simulink library "inp"  (R2021b)
settings: Solver=VariableStepAuto  StartTime=0.0  StopTime=10.0  RelTol=1e-3
undefined symbols (not defined in the file): C_TASK_5MS_S, FALSE, KINP_AcoreReadyToSlp_flg_ovrdflg, KINP_AcoreReadyToSlp_flg_ovrdval, KINP_AllowMovThd_OTA_enum_ovrdflg, KINP_AllowMovThd_OTA_enum_ovrdval, KINP_APSAngleTarget_Deg_ovrdflg, KINP_APSAngleTarget_Deg_ovrdval, KINP_APSDecReq_mps2_ovrdflg, KINP_APSDecReq_mps2_ovrdval, KINP_APSDecReqA_flg_ovrdflg, KINP_APSDecReqA_flg_ovrdval, KINP_APSDFLL_cm_ovrdflg, KINP_APSDFLL_cm_ovrdval, KINP_APSDFLR_cm_ovrdflg, KINP_APSDFLR_cm_ovrdval, KINP_APSDRLL_cm_ovrdflg, KINP_APSDRLL_cm_ovrdval, KINP_APSDRLR_cm_ovrdflg, KINP_APSDRLR_cm_ovrdval, KINP_APSExitCondition_enum_ovrdflg, KINP_APSExitCondition_enum_ovrdval, KINP_APSHWVer_enum_ovrdflg, KINP_APSHWVer_enum_ovrdval, KINP_APSProgressPCT_pct_ovrdflg, KINP_APSProgressPCT_pct_ovrdval, KINP_APSReq_enum_ovrdflg, KINP_APSReq_enum_ovrdval, KINP_APSRQDisplay_enum_ovrdflg, KINP_APSRQDisplay_enum_ovrdval, KINP_APSRqEPASCtrl_flg_ovrdflg, KINP_APSRqEPASCtrl_flg_ovrdval, KINP_APSShiftPosnReq_enum_ovrdval, KINP_APSShiftPosnReq_enum_ovrflg, KINP_APSSpeedCMD_kph_ovrdval, KINP_APSSpeedCMD_kph_ovrflg, KINP_APSStaSystem_enum_ovrdflg, KINP_APSStaSystem_enum_ovrdval, KINP_APSSWVer_enum_ovrdflg, KINP_APSSWVer_enum_ovrdval, KINP_APSVMCReqA_flg_ovrdval, KINP_APSVMCReqA_flg_ovrflg, KINP_APSVRqEPASCtrl_flg_ovrdflg, KINP_APSVRqEPASCtrl_flg_ovrdval, KINP_AuxBattVolmV_mV_ovrdflg, KINP_AuxBattVolmV_mV_ovrdval, KINP_CAASSta_enum_ovrdflg, KINP_CAASSta_enum_ovrdval, KINP_CAASVMCReqA_flg_ovrdval, KINP_CAASVMCReqA_flg_ovrflg, KINP_Chime_enum_ovrdflg, KINP_Chime_enum_ovrdval, KINP_ClearDTCcmd_flg_ovrdflg, KINP_ClearDTCcmd_flg_ovrdval, KINP_EvccAplusPwrUpReq_flg_ovrdflg, KINP_EvccAplusPwrUpReq_flg_ovrdval, KINP_LFID_raw_ovrdval, KINP_LFID_raw_ovrflg, KINP_LRID_raw_ovrdval, KINP_MemOffsetAccX_raw16_ovrdflg ... (+118)
libraries: FVT_lib x595, hcu_lib x1
(part 15 of 27)

== system inp/INP/CAN2/SignalCheck/IVI6 ==
  BHAL_outputs : Inport
  inp_CanValid_bus : Inport  Port=2
  IVILocatedSTA : FVT_lib/inp/can_signal_template  SystemSampleTime=-1  VariantActivationTime=update diagram  Latency=0  AutoFrameSizeCalculation=off
      link override defval: Value=KINP_IVILocatedSTA_enum_defval
      link override fftdec: Value=KINP_IVILocatedSTA_enum_fftdec
      link override fftinc: Value=KINP_IVILocatedSTA_enum_fftinc
      link override fftlim: Value=KINP_IVILocatedSTA_enum_fftlim
      link override invalid: Value=KINP_IVILocatedSTA_enum_invalid
      link override ovrdflg: Value=KINP_IVILocatedSTA_enum_ovrdflg
      link override ovrdval: Value=KINP_IVILocatedSTA_enum_ovrdval
      link override setvalid: Value=KINP_IVILocatedSTA_enum_setvalid
      link override srvcflg: Value=KINP_IVILocatedSTA_enum_srvcflg
      link override srvcval: Value=KINP_IVILocatedSTA_enum_srvcval
  IVITimeCheck : FVT_lib/inp/can_signal_template  SystemSampleTime=-1  VariantActivationTime=update diagram  Latency=0  AutoFrameSizeCalculation=off
      link override defval: Value=KINP_IVITimeCheck_enum_defval
      link override fftdec: Value=KINP_IVITimeCheck_enum_fftdec
      link override fftinc: Value=KINP_IVITimeCheck_enum_fftinc
      link override fftlim: Value=KINP_IVITimeCheck_enum_fftlim
      link override invalid: Value=KINP_IVITimeCheck_enum_invalid
      link override ovrdflg: Value=KINP_IVITimeCheck_enum_ovrdflg
      link override ovrdval: Value=KINP_IVITimeCheck_enum_ovrdval
      link override setvalid: Value=KINP_IVITimeCheck_enum_setvalid
      link override srvcflg: Value=KINP_IVITimeCheck_enum_srvcflg
      link override srvcval: Value=KINP_IVITimeCheck_enum_srvcval
  IVITimeDay : FVT_lib/inp/can_signal_template  SystemSampleTime=-1  VariantActivationTime=update diagram  Latency=0  AutoFrameSizeCalculation=off
      link override defval: Value=KINP_IVITimeDay_DAY_defval
      link override fftdec: Value=KINP_IVITimeDay_DAY_fftdec
      link override fftinc: Value=KINP_IVITimeDay_DAY_fftinc
      link override fftlim: Value=KINP_IVITimeDay_DAY_fftlim
      link override invalid: Value=KINP_IVITimeDay_DAY_invalid
      link override ovrdflg: Value=KINP_IVITimeDay_DAY_ovrdflg
      link override ovrdval: Value=KINP_IVITimeDay_DAY_ovrdval
      link override setvalid: Value=KINP_IVITimeDay_DAY_setvalid
      link override srvcflg: Value=KINP_IVITimeDay_DAY_srvcflg
      link override srvcval: Value=KINP_IVITimeDay_DAY_srvcval
  IVITimeHour : FVT_lib/inp/can_signal_template  SystemSampleTime=-1  VariantActivationTime=update diagram  Latency=0  AutoFrameSizeCalculation=off
      link override defval: Value=KINP_IVITimeHour_hr_defval
      link override fftdec: Value=KINP_IVITimeHour_hr_fftdec
      link override fftinc: Value=KINP_IVITimeHour_hr_fftinc
      link override fftlim: Value=KINP_IVITimeHour_hr_fftlim
      link override invalid: Value=KINP_IVITimeHour_hr_invalid
      link override ovrdflg: Value=KINP_IVITimeHour_hr_ovrdflg
      link override ovrdval: Value=KINP_IVITimeHour_hr_ovrdval
      link override setvalid: Value=KINP_IVITimeHour_hr_setvalid
      link override srvcflg: Value=KINP_IVITimeHour_hr_srvcflg
      link override srvcval: Value=KINP_IVITimeHour_hr_srvcval
  IVITimeMinute : FVT_lib/inp/can_signal_template  SystemSampleTime=-1  VariantActivationTime=update diagram  Latency=0  AutoFrameSizeCalculation=off
      link override defval: Value=KINP_IVITimeMinute_min_defval
      link override fftdec: Value=KINP_IVITimeMinute_min_fftdec
      link override fftinc: Value=KINP_IVITimeMinute_min_fftinc
      link override fftlim: Value=KINP_IVITimeMinute_min_fftlim
      link override invalid: Value=KINP_IVITimeMinute_min_invalid
      link override ovrdflg: Value=KINP_IVITimeMinute_min_ovrdflg
      link override ovrdval: Value=KINP_IVITimeMinute_min_ovrdval
      link override setvalid: Value=KINP_IVITimeMinute_min_setvalid
      link override srvcflg: Value=KINP_IVITimeMinute_min_srvcflg
      link override srvcval: Value=KINP_IVITimeMinute_min_srvcval
  IVITimeMonth : FVT_lib/inp/can_signal_template  SystemSampleTime=-1  VariantActivationTime=update diagram  Latency=0  AutoFrameSizeCalculation=off
      link override defval: Value=KINP_IVITimeMonth_MONTH_defval
      link override fftdec: Value=KINP_IVITimeMonth_MONTH_fftdec
      link override fftinc: Value=KINP_IVITimeMonth_MONTH_fftinc
      link override fftlim: Value=KINP_IVITimeMonth_MONTH_fftlim
      link override invalid: Value=KINP_IVITimeMonth_MONTH_invalid
      link override ovrdflg: Value=KINP_IVITimeMonth_MONTH_ovrdflg
      link override ovrdval: Value=KINP_IVITimeMonth_MONTH_ovrdval
      link override setvalid: Value=KINP_IVITimeMonth_MONTH_setvalid
      link override srvcflg: Value=KINP_IVITimeMonth_MONTH_srvcflg
      link override srvcval: Value=KINP_IVITimeMonth_MONTH_srvcval
  IVITimeSecond : FVT_lib/inp/can_signal_template  SystemSampleTime=-1  VariantActivationTime=update diagram  Latency=0  AutoFrameSizeCalculation=off
      link override defval: Value=KINP_IVITimeSecond_s_defval
      link override fftdec: Value=KINP_IVITimeSecond_s_fftdec
      link override fftinc: Value=KINP_IVITimeSecond_s_fftinc
      link override fftlim: Value=KINP_IVITimeSecond_s_fftlim
      link override invalid: Value=KINP_IVITimeSecond_s_invalid
      link override ovrdflg: Value=KINP_IVITimeSecond_s_ovrdflg
      link override ovrdval: Value=KINP_IVITimeSecond_s_ovrdval
      link override setvalid: Value=KINP_IVITimeSecond_s_setvalid
      link override srvcflg: Value=KINP_IVITimeSecond_s_srvcflg
      link override srvcval: Value=KINP_IVITimeSecond_s_srvcval
  IVITimeYear : FVT_lib/inp/can_signal_template  SystemSampleTime=-1  VariantActivationTime=update diagram  Latency=0  AutoFrameSizeCalculation=off
      link override defval: Value=KINP_IVITimeYear_YEAR_defval
      link override fftdec: Value=KINP_IVITimeYear_YEAR_fftdec
      link override fftinc: Value=KINP_IVITimeYear_YEAR_fftinc
      link override fftlim: Value=KINP_IVITimeYear_YEAR_fftlim
      link override invalid: Value=KINP_IVITimeYear_YEAR_invalid
      link override ovrdflg: Value=KINP_IVITimeYear_YEAR_ovrdflg
      link override ovrdval: Value=KINP_IVITimeYear_YEAR_ovrdval
      link override setvalid: Value=KINP_IVITimeYear_YEAR_setvalid
      link override srvcflg: Value=KINP_IVITimeYear_YEAR_srvcflg
      link override srvcval: Value=KINP_IVITimeYear_YEAR_srvcval
  Terminator_{1..8} (8 alike) : Terminator
  True_VHAL_IVILocatedSTA_enum : Constant  Value=TRUE  OutDataTypeStr=boolean
  True_VHAL_IVITimeCheck_enum : Constant  Value=TRUE  OutDataTypeStr=boolean
  True_VHAL_IVITimeDay_DAY : Constant  Value=TRUE  OutDataTypeStr=boolean
  True_VHAL_IVITimeHour_hr : Constant  Value=TRUE  OutDataTypeStr=boolean
  True_VHAL_IVITimeMinute_min : Constant  Value=TRUE  OutDataTypeStr=boolean
  True_VHAL_IVITimeMonth_MONTH : Constant  Value=TRUE  OutDataTypeStr=boolean
  True_VHAL_IVITimeSecond_s : Constant  Value=TRUE  OutDataTypeStr=boolean
  True_VHAL_IVITimeYear_YEAR : Constant  Value=TRUE  OutDataTypeStr=boolean
  slr1_{1..8} (8 alike) : BusSelector  OutputSignals=VINP_CANMsgValidIVI6_flg
  slr_VHAL_IVILocatedSTA_enum : BusSelector  OutputSignals=VHAL_IVILocatedSTA_enum
  slr_VHAL_IVITimeCheck_enum : BusSelector  OutputSignals=VHAL_IVITimeCheck_enum
  slr_VHAL_IVITimeDay_DAY : BusSelector  OutputSignals=VHAL_IVITimeDay_DAY
  slr_VHAL_IVITimeHour_hr : BusSelector  OutputSignals=VHAL_IVITimeHour_hr
  slr_VHAL_IVITimeMinute_min : BusSelector  OutputSignals=VHAL_IVITimeMinute_min
  slr_VHAL_IVITimeMonth_MONTH : BusSelector  OutputSignals=VHAL_IVITimeMonth_MONTH
  slr_VHAL_IVITimeSecond_s : BusSelector  OutputSignals=VHAL_IVITimeSecond_s
  slr_VHAL_IVITimeYear_YEAR : BusSelector  OutputSignals=VHAL_IVITimeYear_YEAR
  VINP_IVILocatedSTA_enum : Outport
  VINP_IVITimeCheck_enum : Outport  Port=2
  VINP_IVITimeDay_DAY : Outport  Port=3
  VINP_IVITimeHour_hr : Outport  Port=4
  VINP_IVITimeMinute_min : Outport  Port=5
  VINP_IVITimeMonth_MONTH : Outport  Port=6
  VINP_IVITimeSecond_s : Outport  Port=7
  VINP_IVITimeYear_YEAR : Outport  Port=8
  wires:
  BHAL_outputs/1 -> [BHAL_outputs]
  inp_CanValid_bus/1 -> [inp_CanValid_bus]
  [BHAL_outputs] -> slr_VHAL_IVILocatedSTA_enum/1
  slr_VHAL_IVILocatedSTA_enum/1 -> IVILocatedSTA/1  "<VHAL_IVILocatedSTA_enum>"
  True_VHAL_IVILocatedSTA_enum/1 -> IVILocatedSTA/2
  [inp_CanValid_bus] -> slr1_1/1
  slr1_1/1 -> IVILocatedSTA/3  "<VINP_CANMsgValidIVI6_flg>"
  IVILocatedSTA/1 -> VINP_IVILocatedSTA_enum/1  "VINP_IVILocatedSTA_enum"
  IVILocatedSTA/2 -> Terminator_1/1
  [BHAL_outputs] -> slr_VHAL_IVITimeCheck_enum/1
  slr_VHAL_IVITimeCheck_enum/1 -> IVITimeCheck/1  "<VHAL_IVITimeCheck_enum>"
  True_VHAL_IVITimeCheck_enum/1 -> IVITimeCheck/2
  [inp_CanValid_bus] -> slr1_2/1
  slr1_2/1 -> IVITimeCheck/3  "<VINP_CANMsgValidIVI6_flg>"
  IVITimeCheck/1 -> VINP_IVITimeCheck_enum/1  "VINP_IVITimeCheck_enum"
  IVITimeCheck/2 -> Terminator_2/1
  [BHAL_outputs] -> slr_VHAL_IVITimeDay_DAY/1
  slr_VHAL_IVITimeDay_DAY/1 -> IVITimeDay/1  "<VHAL_IVITimeDay_DAY>"
  True_VHAL_IVITimeDay_DAY/1 -> IVITimeDay/2
  [inp_CanValid_bus] -> slr1_3/1
  slr1_3/1 -> IVITimeDay/3  "<VINP_CANMsgValidIVI6_flg>"
  IVITimeDay/1 -> VINP_IVITimeDay_DAY/1  "VINP_IVITimeDay_DAY"
  IVITimeDay/2 -> Terminator_3/1
  [BHAL_outputs] -> slr_VHAL_IVITimeHour_hr/1
  slr_VHAL_IVITimeHour_hr/1 -> IVITimeHour/1  "<VHAL_IVITimeHour_hr>"
  True_VHAL_IVITimeHour_hr/1 -> IVITimeHour/2
  [inp_CanValid_bus] -> slr1_4/1
  slr1_4/1 -> IVITimeHour/3  "<VINP_CANMsgValidIVI6_flg>"
  IVITimeHour/1 -> VINP_IVITimeHour_hr/1  "VINP_IVITimeHour_hr"
  IVITimeHour/2 -> Terminator_4/1
  [BHAL_outputs] -> slr_VHAL_IVITimeMinute_min/1
  slr_VHAL_IVITimeMinute_min/1 -> IVITimeMinute/1  "<VHAL_IVITimeMinute_min>"
  True_VHAL_IVITimeMinute_min/1 -> IVITimeMinute/2
  [inp_CanValid_bus] -> slr1_5/1
  slr1_5/1 -> IVITimeMinute/3  "<VINP_CANMsgValidIVI6_flg>"
  IVITimeMinute/1 -> VINP_IVITimeMinute_min/1  "VINP_IVITimeMinute_min"
  IVITimeMinute/2 -> Terminator_5/1
  [BHAL_outputs] -> slr_VHAL_IVITimeMonth_MONTH/1
  slr_VHAL_IVITimeMonth_MONTH/1 -> IVITimeMonth/1  "<VHAL_IVITimeMonth_MONTH>"
  True_VHAL_IVITimeMonth_MONTH/1 -> IVITimeMonth/2
  [inp_CanValid_bus] -> slr1_6/1
  slr1_6/1 -> IVITimeMonth/3  "<VINP_CANMsgValidIVI6_flg>"
  IVITimeMonth/1 -> VINP_IVITimeMonth_MONTH/1  "VINP_IVITimeMonth_MONTH"
  IVITimeMonth/2 -> Terminator_6/1
  [BHAL_outputs] -> slr_VHAL_IVITimeSecond_s/1
  slr_VHAL_IVITimeSecond_s/1 -> IVITimeSecond/1  "<VHAL_IVITimeSecond_s>"
  True_VHAL_IVITimeSecond_s/1 -> IVITimeSecond/2
  [inp_CanValid_bus] -> slr1_7/1
  slr1_7/1 -> IVITimeSecond/3  "<VINP_CANMsgValidIVI6_flg>"
  IVITimeSecond/1 -> VINP_IVITimeSecond_s/1  "VINP_IVITimeSecond_s"
  IVITimeSecond/2 -> Terminator_7/1
  [BHAL_outputs] -> slr_VHAL_IVITimeYear_YEAR/1
  slr_VHAL_IVITimeYear_YEAR/1 -> IVITimeYear/1  "<VHAL_IVITimeYear_YEAR>"
  True_VHAL_IVITimeYear_YEAR/1 -> IVITimeYear/2
  [inp_CanValid_bus] -> slr1_8/1
  slr1_8/1 -> IVITimeYear/3  "<VINP_CANMsgValidIVI6_flg>"
  IVITimeYear/1 -> VINP_IVITimeYear_YEAR/1  "VINP_IVITimeYear_YEAR"
  IVITimeYear/2 -> Terminator_8/1

== system inp/INP/CAN2/SignalCheck/METER1 ==
  BHAL_outputs : Inport
  inp_CanValid_bus : Inport  Port=2
  METERKPHCalcu : FVT_lib/inp/can_signal_template  SystemSampleTime=-1  VariantActivationTime=update diagram  Latency=0  AutoFrameSizeCalculation=off
      link override defval: Value=KINP_METERKPHCalcu_kph_defval
      link override fftdec: Value=KINP_METERKPHCalcu_kph_fftdec
      link override fftinc: Value=KINP_METERKPHCalcu_kph_fftinc
      link override fftlim: Value=KINP_METERKPHCalcu_kph_fftlim
      link override invalid: Value=KINP_METERKPHCalcu_kph_invalid
      link override ovrdflg: Value=KINP_METERKPHCalcu_kph_ovrdflg
      link override ovrdval: Value=KINP_METERKPHCalcu_kph_ovrdval
      link override setvalid: Value=KINP_METERKPHCalcu_kph_setvalid
      link override srvcflg: Value=KINP_METERKPHCalcu_kph_srvcflg
      link override srvcval: Value=KINP_METERKPHCalcu_kph_srvcval
  Terminator_1 : Terminator
  True_VHAL_METERKPHCalcu_kph : Constant  Value=TRUE  OutDataTypeStr=boolean
  slr1_1 : BusSelector  OutputSignals=VINP_CANMsgValidMETER1_flg
  slr_VHAL_METERKPHCalcu_kph : BusSelector  OutputSignals=VHAL_METERKPHCalcu_kph
  VINP_METERKPHCalcu_kph : Outport
  wires:
  BHAL_outputs/1 -> [BHAL_outputs]
  inp_CanValid_bus/1 -> [inp_CanValid_bus]
  [BHAL_outputs] -> slr_VHAL_METERKPHCalcu_kph/1
  slr_VHAL_METERKPHCalcu_kph/1 -> METERKPHCalcu/1  "<VHAL_METERKPHCalcu_kph>"
  True_VHAL_METERKPHCalcu_kph/1 -> METERKPHCalcu/2
  [inp_CanValid_bus] -> slr1_1/1
  slr1_1/1 -> METERKPHCalcu/3  "<VINP_CANMsgValidMETER1_flg>"
  METERKPHCalcu/1 -> VINP_METERKPHCalcu_kph/1  "VINP_METERKPHCalcu_kph"
  METERKPHCalcu/2 -> Terminator_1/1

== system inp/INP/CAN3/SignalCheck/BMS1 ==
  BHAL_outputs : Inport
  inp_CanValid_bus : Inport  Port=2
  BMS1CSErr : FVT_lib/inp/can_signal_template  SystemSampleTime=-1  VariantActivationTime=update diagram  Latency=0  AutoFrameSizeCalculation=off
      link override defval: Value=KINP_BMS1CSErr_flg_defval
      link override fftdec: Value=KINP_BMS1CSErr_flg_fftdec
      link override fftinc: Value=KINP_BMS1CSErr_flg_fftinc
      link override fftlim: Value=KINP_BMS1CSErr_flg_fftlim
      link override invalid: Value=KINP_BMS1CSErr_flg_invalid
      link override ovrdflg: Value=KINP_BMS1CSErr_flg_ovrdflg
      link override ovrdval: Value=KINP_BMS1CSErr_flg_ovrdval
      link override setvalid: Value=KINP_BMS1CSErr_flg_setvalid
      link override srvcflg: Value=KINP_BMS1CSErr_flg_srvcflg
      link override srvcval: Value=KINP_BMS1CSErr_flg_srvcval
  BMS1RCErr : FVT_lib/inp/can_signal_template  SystemSampleTime=-1  VariantActivationTime=update diagram  Latency=0  AutoFrameSizeCalculation=off
      link override defval: Value=KINP_BMS1RCErr_flg_defval
      link override fftdec: Value=KINP_BMS1RCErr_flg_fftdec
      link override fftinc: Value=KINP_BMS1RCErr_flg_fftinc
      link override fftlim: Value=KINP_BMS1RCErr_flg_fftlim
      link override invalid: Value=KINP_BMS1RCErr_flg_invalid
      link override ovrdflg: Value=KINP_BMS1RCErr_flg_ovrdflg
      link override ovrdval: Value=KINP_BMS1RCErr_flg_ovrdval
      link override setvalid: Value=KINP_BMS1RCErr_flg_setvalid
      link override srvcflg: Value=KINP_BMS1RCErr_flg_srvcflg
      link override srvcval: Value=KINP_BMS1RCErr_flg_srvcval
  BMSChckSum1 : FVT_lib/inp/can_signal_template  SystemSampleTime=-1  VariantActivationTime=update diagram  Latency=0  AutoFrameSizeCalculation=off
      link override defval: Value=KINP_BMSChckSum1_enum_defval
      link override fftdec: Value=KINP_BMSChckSum1_enum_fftdec
      link override fftinc: Value=KINP_BMSChckSum1_enum_fftinc
      link override fftlim: Value=KINP_BMSChckSum1_enum_fftlim
      link override invalid: Value=KINP_BMSChckSum1_enum_invalid
      link override ovrdflg: Value=KINP_BMSChckSum1_enum_ovrdflg
      link override ovrdval: Value=KINP_BMSChckSum1_enum_ovrdval
      link override setvalid: Value=KINP_BMSChckSum1_enum_setvalid
      link override srvcflg: Value=KINP_BMSChckSum1_enum_srvcflg
      link override srvcval: Value=KINP_BMSChckSum1_enum_srvcval
  BMSRolCnct1 : FVT_lib/inp/can_signal_template  SystemSampleTime=-1  VariantActivationTime=update diagram  Latency=0  AutoFrameSizeCalculation=off
      link override defval: Value=KINP_BMSRolCnct1_enum_defval
      link override fftdec: Value=KINP_BMSRolCnct1_enum_fftdec
      link override fftinc: Value=KINP_BMSRolCnct1_enum_fftinc
      link override fftlim: Value=KINP_BMSRolCnct1_enum_fftlim
      link override invalid: Value=KINP_BMSRolCnct1_enum_invalid
      link override ovrdflg: Value=KINP_BMSRolCnct1_enum_ovrdflg
      link override ovrdval: Value=KINP_BMSRolCnct1_enum_ovrdval
      link override setvalid: Value=KINP_BMSRolCnct1_enum_setvalid
      link override srvcflg: Value=KINP_BMSRolCnct1_enum_srvcflg
      link override srvcval: Value=KINP_BMSRolCnct1_enum_srvcval
  HVBPwrAvailChrg : FVT_lib/inp/can_signal_template  SystemSampleTime=-1  VariantActivationTime=update diagram  Latency=0  AutoFrameSizeCalculation=off
      link override defval: Value=KINP_HVBPwrAvailChrg_kW_defval
      link override fftdec: Value=KINP_HVBPwrAvailChrg_kW_fftdec
      link override fftinc: Value=KINP_HVBPwrAvailChrg_kW_fftinc
      link override fftlim: Value=KINP_HVBPwrAvailChrg_kW_fftlim
      link override invalid: Value=KINP_HVBPwrAvailChrg_kW_invalid
      link override ovrdflg: Value=KINP_HVBPwrAvailChrg_kW_ovrdflg
      link override ovrdval: Value=KINP_HVBPwrAvailChrg_kW_ovrdval
      link override setvalid: Value=KINP_HVBPwrAvailChrg_kW_setvalid
      link override srvcflg: Value=KINP_HVBPwrAvailChrg_kW_srvcflg
      link override srvcval: Value=KINP_HVBPwrAvailChrg_kW_srvcval
  HVBPwrAvailChrg30 : FVT_lib/inp/can_signal_template  SystemSampleTime=-1  VariantActivationTime=update diagram  Latency=0  AutoFrameSizeCalculation=off
      link override defval: Value=KINP_HVBPwrAvailChrg30_kW_defval
      link override fftdec: Value=KINP_HVBPwrAvailChrg30_kW_fftdec
      link override fftinc: Value=KINP_HVBPwrAvailChrg30_kW_fftinc
      link override fftlim: Value=KINP_HVBPwrAvailChrg30_kW_fftlim
      link override invalid: Value=KINP_HVBPwrAvailChrg30_kW_invalid
      link override ovrdflg: Value=KINP_HVBPwrAvailChrg30_kW_ovrdflg
      link override ovrdval: Value=KINP_HVBPwrAvailChrg30_kW_ovrdval
      link override setvalid: Value=KINP_HVBPwrAvailChrg30_kW_setvalid
      link override srvcflg: Value=KINP_HVBPwrAvailChrg30_kW_srvcflg
      link override srvcval: Value=KINP_HVBPwrAvailChrg30_kW_srvcval
  HVBPwrAvailChrg60 : FVT_lib/inp/can_signal_template  SystemSampleTime=-1  VariantActivationTime=update diagram  Latency=0  AutoFrameSizeCalculation=off
      link override defval: Value=KINP_HVBPwrAvailChrg60_kW_defval
      link override fftdec: Value=KINP_HVBPwrAvailChrg60_kW_fftdec
      link override fftinc: Value=KINP_HVBPwrAvailChrg60_kW_fftinc
      link override fftlim: Value=KINP_HVBPwrAvailChrg60_kW_fftlim
      link override invalid: Value=KINP_HVBPwrAvailChrg60_kW_invalid
      link override ovrdflg: Value=KINP_HVBPwrAvailChrg60_kW_ovrdflg
      link override ovrdval: Value=KINP_HVBPwrAvailChrg60_kW_ovrdval
      link override setvalid: Value=KINP_HVBPwrAvailChrg60_kW_setvalid
      link override srvcflg: Value=KINP_HVBPwrAvailChrg60_kW_srvcflg
      link override srvcval: Value=KINP_HVBPwrAvailChrg60_kW_srvcval
  HVBPwrAvailDchrg : FVT_lib/inp/can_signal_template  SystemSampleTime=-1  VariantActivationTime=update diagram  Latency=0  AutoFrameSizeCalculation=off
      link override defval: Value=KINP_HVBPwrAvailDchrg_kW_defval
      link override fftdec: Value=KINP_HVBPwrAvailDchrg_kW_fftdec
      link override fftinc: Value=KINP_HVBPwrAvailDchrg_kW_fftinc
      link override fftlim: Value=KINP_HVBPwrAvailDchrg_kW_fftlim
      link override invalid: Value=KINP_HVBPwrAvailDchrg_kW_invalid
      link override ovrdflg: Value=KINP_HVBPwrAvailDchrg_kW_ovrdflg
      link override ovrdval: Value=KINP_HVBPwrAvailDchrg_kW_ovrdval
      link override setvalid: Value=KINP_HVBPwrAvailDchrg_kW_setvalid
      link override srvcflg: Value=KINP_HVBPwrAvailDchrg_kW_srvcflg
      link override srvcval: Value=KINP_HVBPwrAvailDchrg_kW_srvcval
  HVBPwrAvailDchrg30 : FVT_lib/inp/can_signal_template  SystemSampleTime=-1  VariantActivationTime=update diagram  Latency=0  AutoFrameSizeCalculation=off
      link override defval: Value=KINP_HVBPwrAvailDchrg30_kW_defval
      link override fftdec: Value=KINP_HVBPwrAvailDchrg30_kW_fftdec
      link override fftinc: Value=KINP_HVBPwrAvailDchrg30_kW_fftinc
      link override fftlim: Value=KINP_HVBPwrAvailDchrg30_kW_fftlim
      link override invalid: Value=KINP_HVBPwrAvailDchrg30_kW_invalid
      link override ovrdflg: Value=KINP_HVBPwrAvailDchrg30_kW_ovrdflg
      link override ovrdval: Value=KINP_HVBPwrAvailDchrg30_kW_ovrdval
      link override setvalid: Value=KINP_HVBPwrAvailDchrg30_kW_setvalid
      link override srvcflg: Value=KINP_HVBPwrAvailDchrg30_kW_srvcflg
      link override srvcval: Value=KINP_HVBPwrAvailDchrg30_kW_srvcval
  HVBPwrAvailDchrg60 : FVT_lib/inp/can_signal_template  SystemSampleTime=-1  VariantActivationTime=update diagram  Latency=0  AutoFrameSizeCalculation=off
      link override defval: Value=KINP_HVBPwrAvailDchrg60_kW_defval
      link override fftdec: Value=KINP_HVBPwrAvailDchrg60_kW_fftdec
      link override fftinc: Value=KINP_HVBPwrAvailDchrg60_kW_fftinc
      link override fftlim: Value=KINP_HVBPwrAvailDchrg60_kW_fftlim
      link override invalid: Value=KINP_HVBPwrAvailDchrg60_kW_invalid
      link override ovrdflg: Value=KINP_HVBPwrAvailDchrg60_kW_ovrdflg
      link override ovrdval: Value=KINP_HVBPwrAvailDchrg60_kW_ovrdval
      link override setvalid: Value=KINP_HVBPwrAvailDchrg60_kW_setvalid
      link override srvcflg: Value=KINP_HVBPwrAvailDchrg60_kW_srvcflg
      link override srvcval: Value=KINP_HVBPwrAvailDchrg60_kW_srvcval
  Terminator_{1..10} (10 alike) : Terminator
  True_VHAL_BMS1CSErr_flg : Constant  Value=TRUE  OutDataTypeStr=boolean
  True_VHAL_BMS1RCErr_flg : Constant  Value=TRUE  OutDataTypeStr=boolean
  True_VHAL_BMSChckSum1_enum : Constant  Value=TRUE  OutDataTypeStr=boolean
  True_VHAL_BMSRolCnct1_enum : Constant  Value=TRUE  OutDataTypeStr=boolean
  True_VHAL_HVBPwrAvailChrg30_kW : Constant  Value=TRUE  OutDataTypeStr=boolean
  True_VHAL_HVBPwrAvailChrg60_kW : Constant  Value=TRUE  OutDataTypeStr=boolean
  True_VHAL_HVBPwrAvailChrg_kW : Constant  Value=TRUE  OutDataTypeStr=boolean
  True_VHAL_HVBPwrAvailDchrg30_kW : Constant  Value=TRUE  OutDataTypeStr=boolean
  True_VHAL_HVBPwrAvailDchrg60_kW : Constant  Value=TRUE  OutDataTypeStr=boolean
  True_VHAL_HVBPwrAvailDchrg_kW : Constant  Value=TRUE  OutDataTypeStr=boolean
  slr1_{1..10} (10 alike) : BusSelector  OutputSignals=VINP_CANMsgValidBMS1_flg
  slr_VHAL_BMS1CSErr_flg : BusSelector  OutputSignals=VHAL_BMS1CSErr_flg
  slr_VHAL_BMS1RCErr_flg : BusSelector  OutputSignals=VHAL_BMS1RCErr_flg
  slr_VHAL_BMSChckSum1_enum : BusSelector  OutputSignals=VHAL_BMSChckSum1_enum
  slr_VHAL_BMSRolCnct1_enum : BusSelector  OutputSignals=VHAL_BMSRolCnct1_enum
  slr_VHAL_HVBPwrAvailChrg30_kW : BusSelector  OutputSignals=VHAL_HVBPwrAvailChrg30_kW
  slr_VHAL_HVBPwrAvailChrg60_kW : BusSelector  OutputSignals=VHAL_HVBPwrAvailChrg60_kW
  slr_VHAL_HVBPwrAvailChrg_kW : BusSelector  OutputSignals=VHAL_HVBPwrAvailChrg_kW
  slr_VHAL_HVBPwrAvailDchrg30_kW : BusSelector  OutputSignals=VHAL_HVBPwrAvailDchrg30_kW
  slr_VHAL_HVBPwrAvailDchrg60_kW : BusSelector  OutputSignals=VHAL_HVBPwrAvailDchrg60_kW
  slr_VHAL_HVBPwrAvailDchrg_kW : BusSelector  OutputSignals=VHAL_HVBPwrAvailDchrg_kW
  VINP_BMS1CSErr_flg : Outport
  VINP_BMS1RCErr_flg : Outport  Port=2
  VINP_BMSChckSum1_enum : Outport  Port=3
  VINP_BMSRolCnct1_enum : Outport  Port=4
  VINP_HVBPwrAvailChrg_kW : Outport  Port=5
  VINP_HVBPwrAvailChrg30_kW : Outport  Port=6
  VINP_HVBPwrAvailChrg60_kW : Outport  Port=7
  VINP_HVBPwrAvailDchrg_kW : Outport  Port=8
  VINP_HVBPwrAvailDchrg30_kW : Outport  Port=9
  VINP_HVBPwrAvailDchrg60_kW : Outport  Port=10
  wires:
  BHAL_outputs/1 -> [BHAL_outputs]
  inp_CanValid_bus/1 -> [inp_CanValid_bus]
  [BHAL_outputs] -> slr_VHAL_BMS1CSErr_flg/1
  slr_VHAL_BMS1CSErr_flg/1 -> BMS1CSErr/1  "<VHAL_BMS1CSErr_flg>"
  True_VHAL_BMS1CSErr_flg/1 -> BMS1CSErr/2
  [inp_CanValid_bus] -> slr1_1/1
  slr1_1/1 -> BMS1CSErr/3  "<VINP_CANMsgValidBMS1_flg>"
  BMS1CSErr/1 -> VINP_BMS1CSErr_flg/1  "VINP_BMS1CSErr_flg"
  BMS1CSErr/2 -> Terminator_1/1
  [BHAL_outputs] -> slr_VHAL_BMS1RCErr_flg/1
  slr_VHAL_BMS1RCErr_flg/1 -> BMS1RCErr/1  "<VHAL_BMS1RCErr_flg>"
  True_VHAL_BMS1RCErr_flg/1 -> BMS1RCErr/2
  [inp_CanValid_bus] -> slr1_2/1
  slr1_2/1 -> BMS1RCErr/3  "<VINP_CANMsgValidBMS1_flg>"
  BMS1RCErr/1 -> VINP_BMS1RCErr_flg/1  "VINP_BMS1RCErr_flg"
  BMS1RCErr/2 -> Terminator_2/1
  [BHAL_outputs] -> slr_VHAL_BMSChckSum1_enum/1
  slr_VHAL_BMSChckSum1_enum/1 -> BMSChckSum1/1  "<VHAL_BMSChckSum1_enum>"
  True_VHAL_BMSChckSum1_enum/1 -> BMSChckSum1/2
  [inp_CanValid_bus] -> slr1_3/1
  slr1_3/1 -> BMSChckSum1/3  "<VINP_CANMsgValidBMS1_flg>"
  BMSChckSum1/1 -> VINP_BMSChckSum1_enum/1  "VINP_BMSChckSum1_enum"
  BMSChckSum1/2 -> Terminator_3/1
  [BHAL_outputs] -> slr_VHAL_BMSRolCnct1_enum/1
  slr_VHAL_BMSRolCnct1_enum/1 -> BMSRolCnct1/1  "<VHAL_BMSRolCnct1_enum>"
  True_VHAL_BMSRolCnct1_enum/1 -> BMSRolCnct1/2
  [inp_CanValid_bus] -> slr1_4/1
  slr1_4/1 -> BMSRolCnct1/3  "<VINP_CANMsgValidBMS1_flg>"
  BMSRolCnct1/1 -> VINP_BMSRolCnct1_enum/1  "VINP_BMSRolCnct1_enum"
  BMSRolCnct1/2 -> Terminator_4/1
  [BHAL_outputs] -> slr_VHAL_HVBPwrAvailChrg_kW/1
  slr_VHAL_HVBPwrAvailChrg_kW/1 -> HVBPwrAvailChrg/1  "<VHAL_HVBPwrAvailChrg_kW>"
  True_VHAL_HVBPwrAvailChrg_kW/1 -> HVBPwrAvailChrg/2
  [inp_CanValid_bus] -> slr1_5/1
  slr1_5/1 -> HVBPwrAvailChrg/3  "<VINP_CANMsgValidBMS1_flg>"
  HVBPwrAvailChrg/1 -> VINP_HVBPwrAvailChrg_kW/1  "VINP_HVBPwrAvailChrg_kW"
  HVBPwrAvailChrg/2 -> Terminator_5/1
  [BHAL_outputs] -> slr_VHAL_HVBPwrAvailChrg30_kW/1
  slr_VHAL_HVBPwrAvailChrg30_kW/1 -> HVBPwrAvailChrg30/1  "<VHAL_HVBPwrAvailChrg30_kW>"
  True_VHAL_HVBPwrAvailChrg30_kW/1 -> HVBPwrAvailChrg30/2
  [inp_CanValid_bus] -> slr1_6/1
  slr1_6/1 -> HVBPwrAvailChrg30/3  "<VINP_CANMsgValidBMS1_flg>"
  HVBPwrAvailChrg30/1 -> VINP_HVBPwrAvailChrg30_kW/1  "VINP_HVBPwrAvailChrg30_kW"
  HVBPwrAvailChrg30/2 -> Terminator_6/1
  [BHAL_outputs] -> slr_VHAL_HVBPwrAvailChrg60_kW/1
  slr_VHAL_HVBPwrAvailChrg60_kW/1 -> HVBPwrAvailChrg60/1  "<VHAL_HVBPwrAvailChrg60_kW>"
  True_VHAL_HVBPwrAvailChrg60_kW/1 -> HVBPwrAvailChrg60/2
  [inp_CanValid_bus] -> slr1_7/1
  slr1_7/1 -> HVBPwrAvailChrg60/3  "<VINP_CANMsgValidBMS1_flg>"
  HVBPwrAvailChrg60/1 -> VINP_HVBPwrAvailChrg60_kW/1  "VINP_HVBPwrAvailChrg60_kW"
  HVBPwrAvailChrg60/2 -> Terminator_7/1
  [BHAL_outputs] -> slr_VHAL_HVBPwrAvailDchrg_kW/1
  slr_VHAL_HVBPwrAvailDchrg_kW/1 -> HVBPwrAvailDchrg/1  "<VHAL_HVBPwrAvailDchrg_kW>"
  True_VHAL_HVBPwrAvailDchrg_kW/1 -> HVBPwrAvailDchrg/2
  [inp_CanValid_bus] -> slr1_8/1
  slr1_8/1 -> HVBPwrAvailDchrg/3  "<VINP_CANMsgValidBMS1_flg>"
  HVBPwrAvailDchrg/1 -> VINP_HVBPwrAvailDchrg_kW/1  "VINP_HVBPwrAvailDchrg_kW"
  HVBPwrAvailDchrg/2 -> Terminator_8/1
  [BHAL_outputs] -> slr_VHAL_HVBPwrAvailDchrg30_kW/1
  slr_VHAL_HVBPwrAvailDchrg30_kW/1 -> HVBPwrAvailDchrg30/1  "<VHAL_HVBPwrAvailDchrg30_kW>"
  True_VHAL_HVBPwrAvailDchrg30_kW/1 -> HVBPwrAvailDchrg30/2
  [inp_CanValid_bus] -> slr1_9/1
  slr1_9/1 -> HVBPwrAvailDchrg30/3  "<VINP_CANMsgValidBMS1_flg>"
  HVBPwrAvailDchrg30/1 -> VINP_HVBPwrAvailDchrg30_kW/1  "VINP_HVBPwrAvailDchrg30_kW"
  HVBPwrAvailDchrg30/2 -> Terminator_9/1
  [BHAL_outputs] -> slr_VHAL_HVBPwrAvailDchrg60_kW/1
  slr_VHAL_HVBPwrAvailDchrg60_kW/1 -> HVBPwrAvailDchrg60/1  "<VHAL_HVBPwrAvailDchrg60_kW>"
  True_VHAL_HVBPwrAvailDchrg60_kW/1 -> HVBPwrAvailDchrg60/2
  [inp_CanValid_bus] -> slr1_10/1
  slr1_10/1 -> HVBPwrAvailDchrg60/3  "<VINP_CANMsgValidBMS1_flg>"
  HVBPwrAvailDchrg60/1 -> VINP_HVBPwrAvailDchrg60_kW/1  "VINP_HVBPwrAvailDchrg60_kW"
  HVBPwrAvailDchrg60/2 -> Terminator_10/1

== system inp/INP/CAN3/SignalCheck/BMS2 ==
  BHAL_outputs : Inport
  inp_CanValid_bus : Inport  Port=2
  HVInVolt : FVT_lib/inp/can_signal_template  SystemSampleTime=-1  VariantActivationTime=update diagram  Latency=0  AutoFrameSizeCalculation=off
      link override defval: Value=KINP_HVInVolt_V_defval
      link override fftdec: Value=KINP_HVInVolt_V_fftdec
      link override fftinc: Value=KINP_HVInVolt_V_fftinc
      link override fftlim: Value=KINP_HVInVolt_V_fftlim
      link override invalid: Value=KINP_HVInVolt_V_invalid
      link override ovrdflg: Value=KINP_HVInVolt_V_ovrdflg
      link override ovrdval: Value=KINP_HVInVolt_V_ovrdval
      link override setvalid: Value=KINP_HVInVolt_V_setvalid
      link override srvcflg: Value=KINP_HVInVolt_V_srvcflg
      link override srvcval: Value=KINP_HVInVolt_V_srvcval
  LVBattDet12V : FVT_lib/inp/can_signal_template  SystemSampleTime=-1  VariantActivationTime=update diagram  Latency=0  AutoFrameSizeCalculation=off
      link override defval: Value=KINP_LVBattDet12V_V_defval
      link override fftdec: Value=KINP_LVBattDet12V_V_fftdec
      link override fftinc: Value=KINP_LVBattDet12V_V_fftinc
      link override fftlim: Value=KINP_LVBattDet12V_V_fftlim
      link override invalid: Value=KINP_LVBattDet12V_V_invalid
      link override ovrdflg: Value=KINP_LVBattDet12V_V_ovrdflg
      link override ovrdval: Value=KINP_LVBattDet12V_V_ovrdval
      link override setvalid: Value=KINP_LVBattDet12V_V_setvalid
      link override srvcflg: Value=KINP_LVBattDet12V_V_srvcflg
      link override srvcval: Value=KINP_LVBattDet12V_V_srvcval
  OBCDCCurLm : FVT_lib/inp/can_signal_template  SystemSampleTime=-1  VariantActivationTime=update diagram  Latency=0  AutoFrameSizeCalculation=off
      link override defval: Value=KINP_OBCDCCurLm_A_defval
      link override fftdec: Value=KINP_OBCDCCurLm_A_fftdec
      link override fftinc: Value=KINP_OBCDCCurLm_A_fftinc
      link override fftlim: Value=KINP_OBCDCCurLm_A_fftlim
      link override invalid: Value=KINP_OBCDCCurLm_A_invalid
      link override ovrdflg: Value=KINP_OBCDCCurLm_A_ovrdflg
      link override ovrdval: Value=KINP_OBCDCCurLm_A_ovrdval
      link override setvalid: Value=KINP_OBCDCCurLm_A_setvalid
      link override srvcflg: Value=KINP_OBCDCCurLm_A_srvcflg
      link override srvcval: Value=KINP_OBCDCCurLm_A_srvcval
  OBCDCVoltLm : FVT_lib/inp/can_signal_template  SystemSampleTime=-1  VariantActivationTime=update diagram  Latency=0  AutoFrameSizeCalculation=off
      link override defval: Value=KINP_OBCDCVoltLm_V_defval
      link override fftdec: Value=KINP_OBCDCVoltLm_V_fftdec
      link override fftinc: Value=KINP_OBCDCVoltLm_V_fftinc
      link override fftlim: Value=KINP_OBCDCVoltLm_V_fftlim
      link override invalid: Value=KINP_OBCDCVoltLm_V_invalid
      link override ovrdflg: Value=KINP_OBCDCVoltLm_V_ovrdflg
      link override ovrdval: Value=KINP_OBCDCVoltLm_V_ovrdval
      link override setvalid: Value=KINP_OBCDCVoltLm_V_setvalid
      link override srvcflg: Value=KINP_OBCDCVoltLm_V_srvcflg
      link override srvcval: Value=KINP_OBCDCVoltLm_V_srvcval
  Terminator_{1..4} (4 alike) : Terminator
  True_VHAL_HVInVolt_V : Constant  Value=TRUE  OutDataTypeStr=boolean
  True_VHAL_LVBattDet12V_V : Constant  Value=TRUE  OutDataTypeStr=boolean
  True_VHAL_OBCDCCurLm_A : Constant  Value=TRUE  OutDataTypeStr=boolean
  True_VHAL_OBCDCVoltLm_V : Constant  Value=TRUE  OutDataTypeStr=boolean
  slr1_{1..4} (4 alike) : BusSelector  OutputSignals=VINP_CANMsgValidBMS2_flg
  slr_VHAL_HVInVolt_V : BusSelector  OutputSignals=VHAL_HVInVolt_V
  slr_VHAL_LVBattDet12V_V : BusSelector  OutputSignals=VHAL_LVBattDet12V_V
  slr_VHAL_OBCDCCurLm_A : BusSelector  OutputSignals=VHAL_OBCDCCurLm_A
  slr_VHAL_OBCDCVoltLm_V : BusSelector  OutputSignals=VHAL_OBCDCVoltLm_V
  VINP_HVInVolt_V : Outport
  VINP_LVBattDet12V_V : Outport  Port=2
  VINP_OBCDCCurLm_A : Outport  Port=3
  VINP_OBCDCVoltLm_V : Outport  Port=4
  wires:
  BHAL_outputs/1 -> [BHAL_outputs]
  inp_CanValid_bus/1 -> [inp_CanValid_bus]
  [BHAL_outputs] -> slr_VHAL_HVInVolt_V/1
  slr_VHAL_HVInVolt_V/1 -> HVInVolt/1  "<VHAL_HVInVolt_V>"
  True_VHAL_HVInVolt_V/1 -> HVInVolt/2
  [inp_CanValid_bus] -> slr1_1/1
  slr1_1/1 -> HVInVolt/3  "<VINP_CANMsgValidBMS2_flg>"
  HVInVolt/1 -> VINP_HVInVolt_V/1  "VINP_HVInVolt_V"
  HVInVolt/2 -> Terminator_1/1
  [BHAL_outputs] -> slr_VHAL_LVBattDet12V_V/1
  slr_VHAL_LVBattDet12V_V/1 -> LVBattDet12V/1  "<VHAL_LVBattDet12V_V>"
  True_VHAL_LVBattDet12V_V/1 -> LVBattDet12V/2
  [inp_CanValid_bus] -> slr1_2/1
  slr1_2/1 -> LVBattDet12V/3  "<VINP_CANMsgValidBMS2_flg>"
  LVBattDet12V/1 -> VINP_LVBattDet12V_V/1  "VINP_LVBattDet12V_V"
  LVBattDet12V/2 -> Terminator_2/1
  [BHAL_outputs] -> slr_VHAL_OBCDCCurLm_A/1
  slr_VHAL_OBCDCCurLm_A/1 -> OBCDCCurLm/1  "<VHAL_OBCDCCurLm_A>"
  True_VHAL_OBCDCCurLm_A/1 -> OBCDCCurLm/2
  [inp_CanValid_bus] -> slr1_3/1
  slr1_3/1 -> OBCDCCurLm/3  "<VINP_CANMsgValidBMS2_flg>"
  OBCDCCurLm/1 -> VINP_OBCDCCurLm_A/1  "VINP_OBCDCCurLm_A"
  OBCDCCurLm/2 -> Terminator_3/1
  [BHAL_outputs] -> slr_VHAL_OBCDCVoltLm_V/1
  slr_VHAL_OBCDCVoltLm_V/1 -> OBCDCVoltLm/1  "<VHAL_OBCDCVoltLm_V>"
  True_VHAL_OBCDCVoltLm_V/1 -> OBCDCVoltLm/2
  [inp_CanValid_bus] -> slr1_4/1
  slr1_4/1 -> OBCDCVoltLm/3  "<VINP_CANMsgValidBMS2_flg>"
  OBCDCVoltLm/1 -> VINP_OBCDCVoltLm_V/1  "VINP_OBCDCVoltLm_V"
  OBCDCVoltLm/2 -> Terminator_4/1
